simulink model "currentLoopHarness"  (R2025b)
settings: Solver=VariableStepAuto  StartTime=0.0  StopTime=10.0  RelTol=1e-3
libraries: metux_library x1
settings Model: DataDictionary=motorData.sldd  Creator=karadeli  LastModifiedBy=karadeli

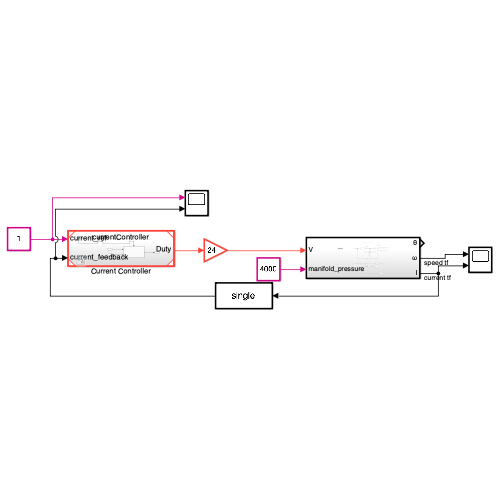
[thumbnail: Simulink's stored preview of the top-level diagram]
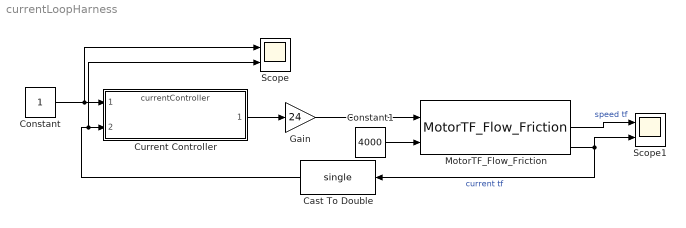
== system currentLoopHarness ==
  Cast To Double : DataTypeConversion  OutDataTypeStr=single  SaturateOnIntegerOverflow=off  RndMeth=Floor
  Constant : Constant  OutDataTypeStr=single
  Constant1 : Constant  Value=4000
  Current Controller : ModelReference  ModelNameDialog=currentController.slx  SimulationMode=Normal  ModelReferenceVersion=1.116
  Gain : Gain  Gain=24
  MotorTF_Flow_Friction : metux_library/MotorTF_Flow_Friction  SystemSampleTime=-1  VariantActivationTime=update diagram  EmptyChoice=off  PassThrough=off  PassThroughVariantControl=(default)  EmptyChoiceVariantControl=(default)  AllowFlexibleInterface=on  Latency=0  AutoFrameSizeCalculation=off
      link override Gain4: Gain=100
  Scope : Scope  NumInputPorts=2
      settings: ActiveDisplayYMinimum=0.99919915944337845  ActiveDisplayYMaximum=1.0000889822840691
  Scope1 : Scope  NumInputPorts=2
      settings: ActiveDisplayYMinimum=-83.091442926080418  ActiveDisplayYMaximum=83.091442926362177
  wires:
  Current Controller/1 -> Gain/1
  Gain/1 -> MotorTF_Flow_Friction/1
  Constant/1 -> Scope/1, Current Controller/1
  MotorTF_Flow_Friction/3 -> Cast To Double/1, Scope1/2  "current tf"
  Cast To Double/1 -> Scope/2, Current Controller/2
  MotorTF_Flow_Friction/2 -> Scope1/1  "speed tf"
  Constant1/1 -> MotorTF_Flow_Friction/2
